simulink model "Lab1_1"  (R2024b)
settings: Solver=VariableStepAuto  StartTime=0.0  StopTime=10.0  RelTol=1e-3
libraries: stm32f4xxblockslib x2
settings Model: STM32="{\"AnalogInput\":{\"ID\":\"Lab1_1:1\"},\"DigitalPortRead\":{\"ID\":\"Lab1_1:8\"}}"  Creator=ASUS  LastModifiedBy=ASUS

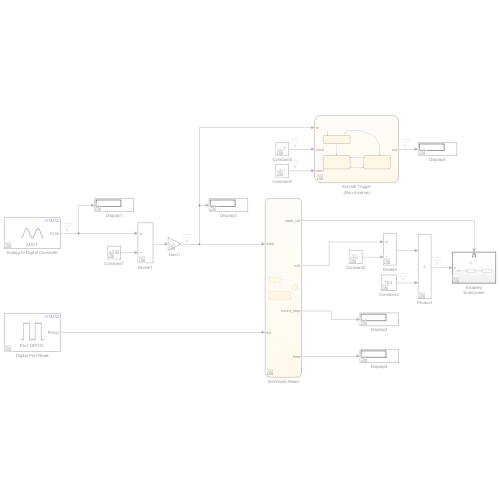
[thumbnail: Simulink's stored preview of the top-level diagram]
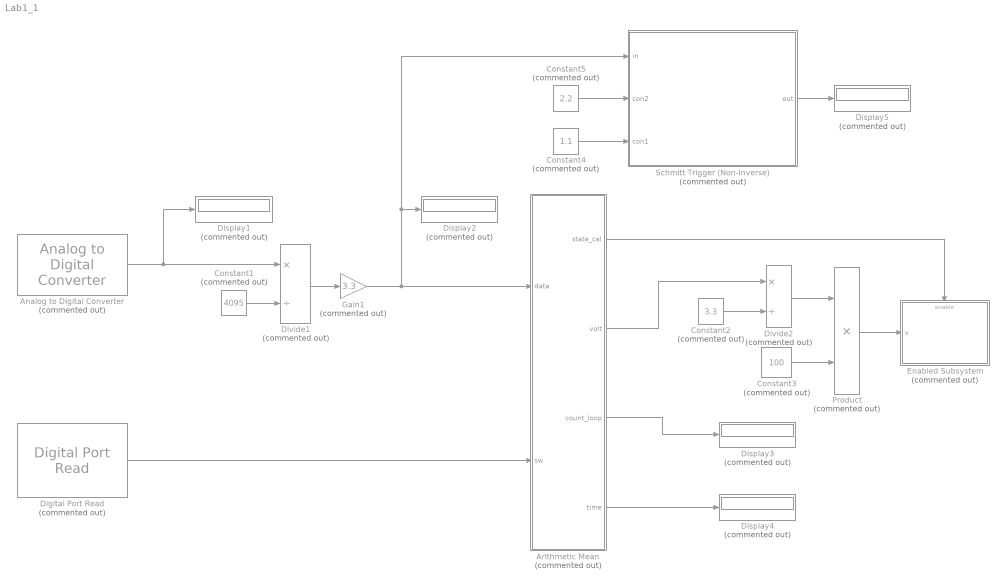
== system Lab1_1 ==
  Analog to Digital Converter : stm32f4xxblockslib/Analog to Digital Converter  Commented=on  ADCModule=ADC1  ConversionGroup=Regular  TriggerMode=Trigger and read  NumberOfConversions=1  EnableBufferConv=off  BufferLength=1  OutputStatus=off  SampleTime=-1  EnableSimPort=off  hoistedMaskSrc=ECSoC/ECSimCodegen/Analog to Digital Converter
  Arithmetic Mean : Stateflow chart  Commented=on  TreatAsAtomicUnit=on
      settings: PortSchema="{\"entries\":[{\"content\":{\"sides\":[{\"content\":{\"connectorIds\":[\"In2\",\"In1\"]},\"type\":\"ConnectorPlacement.EquallySpacedRectSide\",\"uuid\":\"35d75dd1-7445-4d4a-b8fe-26ed95a9a6b8\"},{\"content\":{\"connectorIds\":[\"Out2\",\"Out3\",\"Out4\",\"Out1\"],\"side\":\"RIGHT\"},\"type\":\"ConnectorPlacement.EquallySpacedRectSide\",\"uuid\":\"b4f8c003-30bf-4716-9840-06738554497d\"},{\"content\":{\"side\":\"TOP\"},\"type\":\"ConnectorPlacement.EquallySpacedRectSide\",\"uuid\":\"cf516399-e2a7-4cee-9ef3-409cd0d6a689\"}]},\"type\":\"ConnectorPlacement.EquallySpacedConnector\",\"uuid\":\"7b96adef-8831-434e-9917-44e023cba094\"}],\"packageUris\":[\"http://schema.mathworks.com/mf0/Connector/R2020b\"],\"version\":\"1.0\"}"
  Constant1 : Constant  Commented=on  Value=4095
  Constant2 : Constant  Commented=on  Value=3.3
  Constant3 : Constant  Commented=on  Value=100
  Constant4 : Constant  Commented=on  Value=1.1
  Constant5 : Constant  Commented=on  Value=2.2
  Digital Port Read : stm32f4xxblockslib/Digital Port Read  Commented=on  PortName=GPIOC  PinNumber=13  ReadOperation=on  IOAsArray=on  SampleTime=-1  EnableSimPort=off  hoistedMaskSrc=ECSoC/ECSimCodegen/Digital Port Read
      settings: LibrarySourceBlock=stm32g4xxblockslib/Digital Port Read
  Display{1..5} (5 alike) : Display  Commented=on
  Divide1 : Product  Commented=on  Inputs=*/
  Divide2 : Product  Commented=on  Inputs=*/
  Enabled Subsystem : Subsystem  Commented=on  TreatAsAtomicUnit=on
  Gain1 : Gain  Commented=on  Gain=3.3
  Product : Product  Commented=on
  Schmitt Trigger (Non-Inverse) : Stateflow chart  Commented=on  TreatAsAtomicUnit=on
  wires:
  Divide1/1 -> Gain1/1
  Constant1/1 -> Divide1/2
  Product/1 -> Enabled Subsystem/1(v)
  Digital Port Read/1 -> Arithmetic Mean/1(sw)
  Schmitt Trigger (Non-Inverse)/1(out) -> Display5/1
  Constant4/1 -> Schmitt Trigger (Non-Inverse)/3(con1)
  Analog to Digital Converter/1 -> Divide1/1, Display1/1
  Gain1/1 -> Display2/1, Schmitt Trigger (Non-Inverse)/1(in), Arithmetic Mean/2(data)
  Arithmetic Mean/1(time) -> Display4/1
  Constant5/1 -> Schmitt Trigger (Non-Inverse)/2(con2)
  Arithmetic Mean/4(count_loop) -> Display3/1
  Constant2/1 -> Divide2/2
  Constant3/1 -> Product/2
  Divide2/1 -> Product/1
  Arithmetic Mean/3(volt) -> Divide2/1
  Arithmetic Mean/2(state_cal) -> Enabled Subsystem/Enable

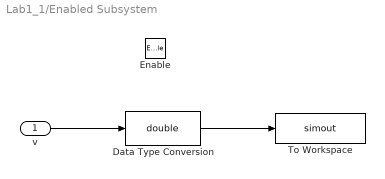
== system Lab1_1/Enabled Subsystem ==
  v : Inport
  Enable : EnablePort
  Data Type Conversion : DataTypeConversion  OutDataTypeStr=double  SaturateOnIntegerOverflow=off  RndMeth=Floor
  To Workspace : ToWorkspace  VariableName=simout  SampleTime=-1
      settings: Save2DSignal=2-D array (concatenate along first dimension)
  wires:
  v/1 -> Data Type Conversion/1
  Data Type Conversion/1 -> To Workspace/1

== stateflow chart Lab1_1/Arithmetic Mean ==
  state Initial
    volt ;
    time = 0;
    state_cal = 0;
    count_loop=0;
  state StopCount
    entry:
    state_cal = 1
  state CountData
    entry:
    volt = data - data;
    during:
    volt = volt + data
    count_loop=count_loop+1
    time=time+0.002
    exit:
    volt = volt/500;
  (default) -> Initial
  StopCount -> Initial
  Initial -> CountData : [sw==1]
  CountData -> StopCount : [time>=1]
  data: sw input; data input; time output; state_cal output; volt output; count_loop output

== stateflow chart Lab1_1/Schmitt Trigger (Non-Inverse) ==
  state Initial_
    out = 0;
  state low1
    entry:
    out=0
  state high
    entry:
    out=1
  Initial_ -> high [order 2] : [in >= con2]
  (default) -> Initial_
  Initial_ -> low1 [order 1] : [in <= con1]
  high -> low1 : [in < con1]
  low1 -> high : [in > con2]
  data: in input; out output; con2 input double; con1 input double
